simulink model "Plant"  (R2021b)
settings: Solver=VariableStepAuto  StartTime=0.0  StopTime=10.0  RelTol=1e-3
model workspace (MAT data in the model file):
  Ax = 0.000556
  Ay = 0.000556
  Az = 0.000635
  Ixx = 0.0075
  Iyy = 0.0075
  Izz = 0.013
  Jr = 6e-05
  b = 3.13e-05
  d = 7.5e-07
  g = 9.81
  l = 0.23
  m = 0.65
settings Model: Creator=aakas  LastModifiedBy=aakas

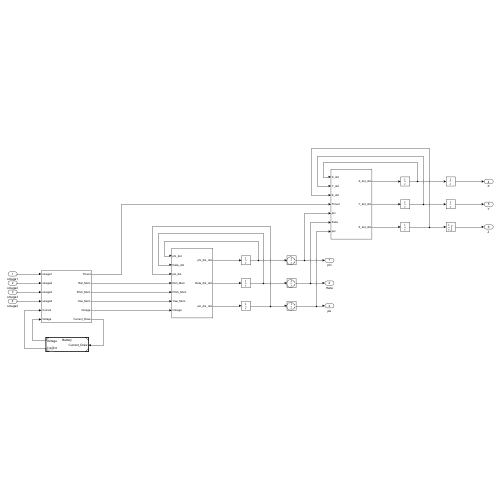
[thumbnail: Simulink's stored preview of the top-level diagram]
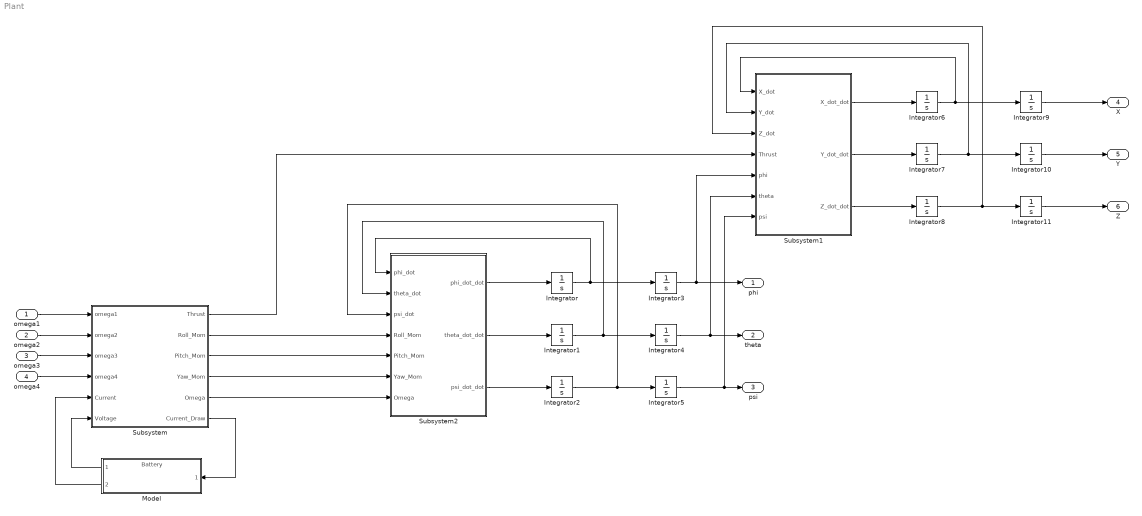
== system Plant ==
  omega1 : Inport
  omega2 : Inport  Port=2
  omega3 : Inport  Port=3
  omega4 : Inport  Port=4
  Integrator{,1..2,6..10} (8 alike) : Integrator
  Integrator11 : Integrator  LimitOutput=on  UpperSaturationLimit=0
  Integrator3 : Integrator  WrapState=on
  Integrator4 : Integrator  WrapState=on
  Integrator5 : Integrator  WrapState=on
  Model : ModelReference  ModelNameDialog=Battery.slx  SimulationMode=Normal  ModelReferenceVersion=1.8
  Subsystem : Subsystem
  Subsystem1 : Subsystem
  Subsystem2 : Subsystem
  phi : Outport
  theta : Outport  Port=2
  psi : Outport  Port=3
  X : Outport  Port=4
  Y : Outport  Port=5
  Z : Outport  Port=6
  wires:
  omega1/1 -> Subsystem/1(omega1)
  omega2/1 -> Subsystem/2(omega2)
  omega3/1 -> Subsystem/3(omega3)
  omega4/1 -> Subsystem/4(omega4)
  Integrator/1 -> Integrator3/1, Subsystem2/1(phi_dot)
  Integrator2/1 -> Subsystem2/3(psi_dot), Integrator5/1
  Integrator3/1 -> Subsystem1/5(phi), phi/1
  Integrator4/1 -> Subsystem1/6(theta), theta/1
  Integrator5/1 -> Subsystem1/7(psi), psi/1
  Integrator1/1 -> Subsystem2/2(theta_dot), Integrator4/1
  Subsystem/2(Roll_Mom) -> Subsystem2/4(Roll_Mom)
  Subsystem/3(Pitch_Mom) -> Subsystem2/5(Pitch_Mom)
  Subsystem/4(Yaw_Mom) -> Subsystem2/6(Yaw_Mom)
  Subsystem/5(Omega) -> Subsystem2/7(Omega)
  Subsystem2/1(phi_dot_dot) -> Integrator/1
  Subsystem2/2(theta_dot_dot) -> Integrator1/1
  Subsystem2/3(psi_dot_dot) -> Integrator2/1
  Integrator6/1 -> Integrator9/1, Subsystem1/1(X_dot)
  Integrator10/1 -> Y/1
  Integrator7/1 -> Subsystem1/2(Y_dot), Integrator10/1
  Integrator11/1 -> Z/1
  Subsystem1/2(Y_dot_dot) -> Integrator7/1
  Subsystem1/3(Z_dot_dot) -> Integrator8/1
  Subsystem1/1(X_dot_dot) -> Integrator6/1
  Integrator9/1 -> X/1
  Integrator8/1 -> Subsystem1/3(Z_dot), Integrator11/1
  Subsystem/1(Thrust) -> Subsystem1/4(Thrust)
  Subsystem/6(Current_Draw) -> Model/1
  Model/1 -> Subsystem/6(Voltage)
  Model/2 -> Subsystem/5(Current)

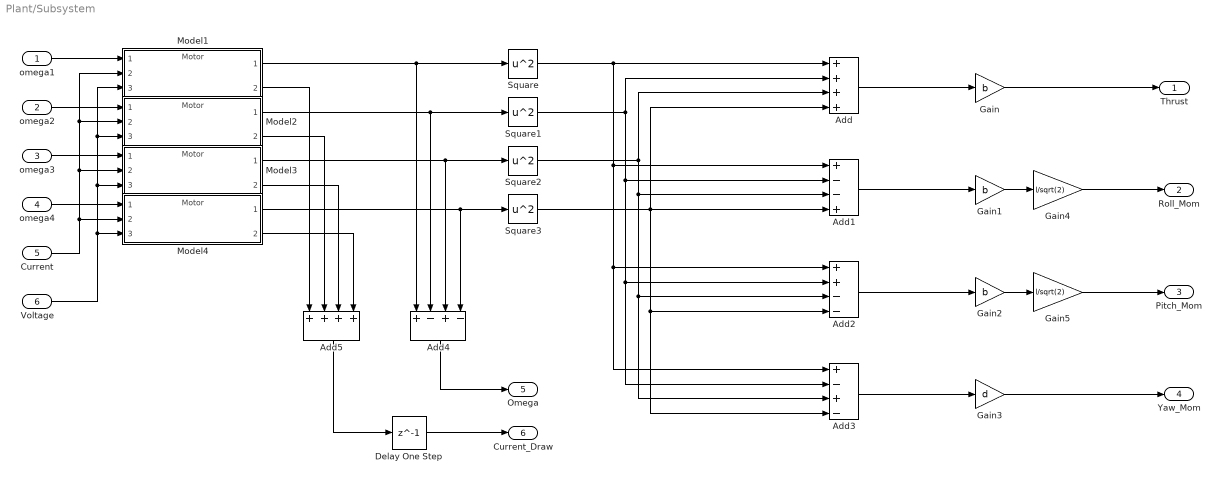
== system Plant/Subsystem ==
  omega1 : Inport
  omega2 : Inport  Port=2
  omega3 : Inport  Port=3
  omega4 : Inport  Port=4
  Current : Inport  Port=5
  Voltage : Inport  Port=6
  Add : Sum  Inputs=++++
  Add1 : Sum  Inputs=+--+
  Add2 : Sum  Inputs=++--
  Add3 : Sum  Inputs=+-+-
  Add4 : Sum  Inputs=+-+-
  Add5 : Sum  Inputs=++++
  Delay One Step : Delay  DelayLength=1
  Gain : Gain  Gain=b
  Gain1 : Gain  Gain=b
  Gain2 : Gain  Gain=b
  Gain3 : Gain  Gain=d
  Gain4 : Gain  Gain=l/sqrt(2)
  Gain5 : Gain  Gain=l/sqrt(2)
  Model{1..4} (4 alike) : ModelReference  ModelNameDialog=Motor.slx  SimulationMode=Normal  ModelReferenceVersion=1.6
  Square{,1..3} (4 alike) : Math  Operator=square  SaturateOnIntegerOverflow=on
  Thrust : Outport
  Roll_Mom : Outport  Port=2
  Pitch_Mom : Outport  Port=3
  Yaw_Mom : Outport  Port=4
  Omega : Outport  Port=5
  Current_Draw : Outport  Port=6
  wires:
  Add2/1 -> Gain2/1
  Model3/1 -> Add4/3, Square2/1
  Model4/1 -> Add4/4, Square3/1
  Add3/1 -> Gain3/1
  Gain2/1 -> Gain5/1
  Square2/1 -> Add3/3, Add2/3, Add1/3, Add/3
  Square3/1 -> Add3/4, Add2/4, Add1/4, Add/4
  Model2/1 -> Add4/2, Square1/1
  Add4/1 -> Omega/1
  Gain4/1 -> Roll_Mom/1
  Gain1/1 -> Gain4/1
  Model1/1 -> Add4/1, Square/1
  Square1/1 -> Add1/2, Add3/2, Add2/2, Add/2
  Gain3/1 -> Yaw_Mom/1
  Square/1 -> Add1/1, Add2/1, Add3/1, Add/1
  Add1/1 -> Gain1/1
  Add/1 -> Gain/1
  Gain/1 -> Thrust/1
  Gain5/1 -> Pitch_Mom/1
  omega1/1 -> Model1/1
  omega2/1 -> Model2/1
  omega3/1 -> Model3/1
  omega4/1 -> Model4/1
  Model1/2 -> Add5/1
  Model2/2 -> Add5/2
  Model4/2 -> Add5/4
  Model3/2 -> Add5/3
  Add5/1 -> Delay One Step/1
  Current/1 -> Model4/2, Model3/2, Model2/2, Model1/2
  Voltage/1 -> Model4/3, Model3/3, Model2/3, Model1/3
  Delay One Step/1 -> Current_Draw/1

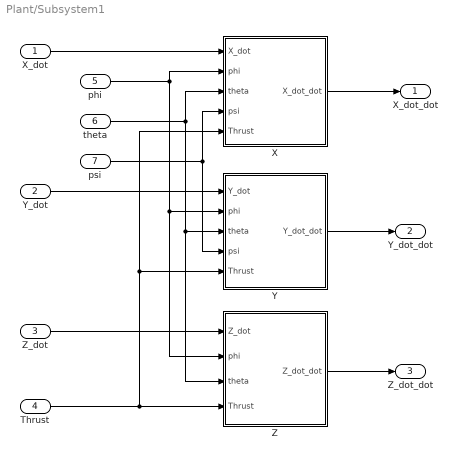
== system Plant/Subsystem1 ==
  X_dot : Inport
  Y_dot : Inport  Port=2
  Z_dot : Inport  Port=3
  Thrust : Inport  Port=4
  phi : Inport  Port=5
  theta : Inport  Port=6
  psi : Inport  Port=7
  X : Subsystem
  Y : Subsystem
  Z : Subsystem
  X_dot_dot : Outport
  Y_dot_dot : Outport  Port=2
  Z_dot_dot : Outport  Port=3
  wires:
  X/1(X_dot_dot) -> X_dot_dot/1
  Z/1(Z_dot_dot) -> Z_dot_dot/1
  Y/1(Y_dot_dot) -> Y_dot_dot/1
  X_dot/1 -> X/1(X_dot)
  Y_dot/1 -> Y/1(Y_dot)
  Z_dot/1 -> Z/1(Z_dot)
  phi/1 -> Z/2(phi), Y/2(phi), X/2(phi)
  theta/1 -> Z/3(theta), Y/3(theta), X/3(theta)
  psi/1 -> Y/4(psi), X/4(psi)
  Thrust/1 -> Z/4(Thrust), Y/5(Thrust), X/5(Thrust)

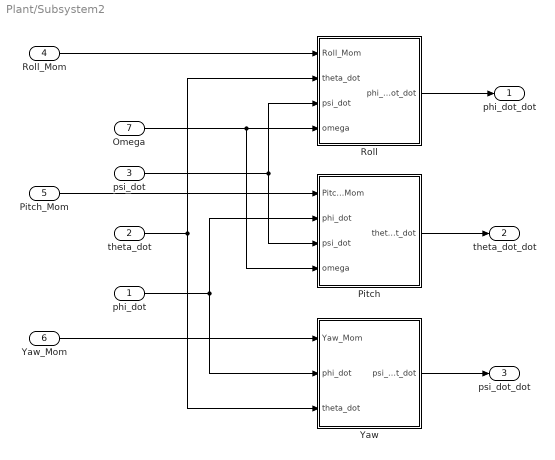
== system Plant/Subsystem2 ==
  phi_dot : Inport
  theta_dot : Inport  Port=2
  psi_dot : Inport  Port=3
  Roll_Mom : Inport  Port=4
  Pitch_Mom : Inport  Port=5
  Yaw_Mom : Inport  Port=6
  Omega : Inport  Port=7
  Pitch : Subsystem
  Roll : Subsystem
  Yaw : Subsystem
  phi_dot_dot : Outport
  theta_dot_dot : Outport  Port=2
  psi_dot_dot : Outport  Port=3
  wires:
  Roll/1(phi_dot_dot) -> phi_dot_dot/1
  Yaw/1(psi_dot_dot) -> psi_dot_dot/1
  Pitch/1(theta_dot_dot) -> theta_dot_dot/1
  Yaw_Mom/1 -> Yaw/1(Yaw_Mom)
  Roll_Mom/1 -> Roll/1(Roll_Mom)
  theta_dot/1 -> Yaw/3(theta_dot), Roll/2(theta_dot)
  Pitch_Mom/1 -> Pitch/1(Pitch_Mom)
  Omega/1 -> Pitch/4(omega), Roll/4(omega)
  psi_dot/1 -> Roll/3(psi_dot), Pitch/3(psi_dot)
  phi_dot/1 -> Yaw/2(phi_dot), Pitch/2(phi_dot)

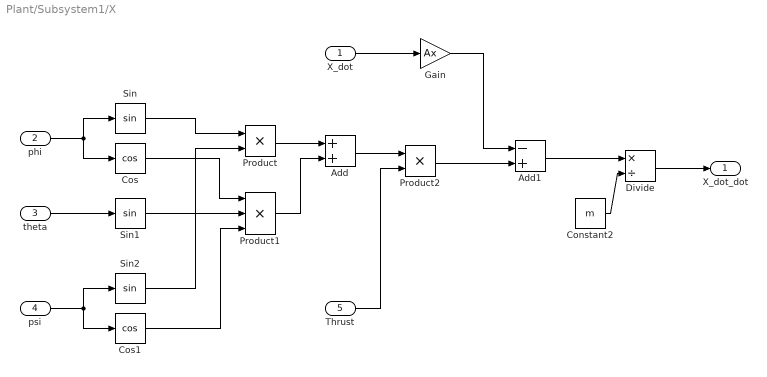
== system Plant/Subsystem1/X ==
  X_dot : Inport
  phi : Inport  Port=2
  theta : Inport  Port=3
  psi : Inport  Port=4
  Thrust : Inport  Port=5
  Add : Sum
  Add1 : Sum  Inputs=-+
  Constant2 : Constant  Value=m
  Cos : Trigonometry  Operator=cos
  Cos1 : Trigonometry  Operator=cos
  Divide : Product  Inputs=*/
  Gain : Gain  Gain=Ax
  Product : Product
  Product1 : Product  Inputs=3
  Product2 : Product
  Sin : Trigonometry
  Sin1 : Trigonometry
  Sin2 : Trigonometry
  X_dot_dot : Outport
  wires:
  Divide/1 -> X_dot_dot/1
  Constant2/1 -> Divide/2
  psi/1 -> Cos1/1, Sin2/1
  phi/1 -> Cos/1, Sin/1
  theta/1 -> Sin1/1
  Sin/1 -> Product/1
  Sin2/1 -> Product/2
  Cos/1 -> Product1/1
  Sin1/1 -> Product1/2
  Cos1/1 -> Product1/3
  Product/1 -> Add/1
  Product1/1 -> Add/2
  Add/1 -> Product2/1
  Thrust/1 -> Product2/2
  Product2/1 -> Add1/2
  Add1/1 -> Divide/1
  X_dot/1 -> Gain/1
  Gain/1 -> Add1/1

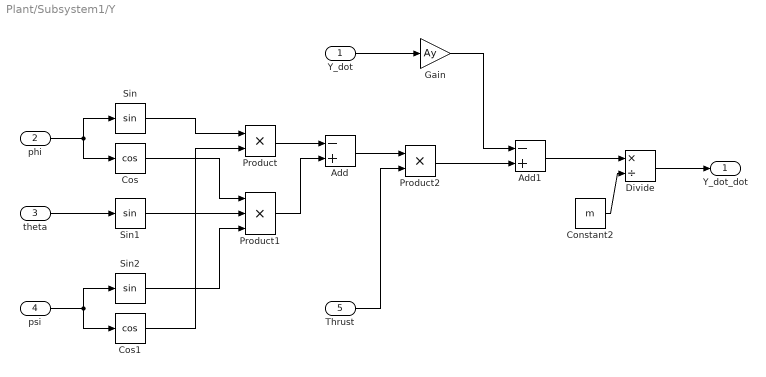
== system Plant/Subsystem1/Y ==
  Y_dot : Inport
  phi : Inport  Port=2
  theta : Inport  Port=3
  psi : Inport  Port=4
  Thrust : Inport  Port=5
  Add : Sum  Inputs=-+
  Add1 : Sum  Inputs=-+
  Constant2 : Constant  Value=m
  Cos : Trigonometry  Operator=cos
  Cos1 : Trigonometry  Operator=cos
  Divide : Product  Inputs=*/
  Gain : Gain  Gain=Ay
  Product : Product
  Product1 : Product  Inputs=3
  Product2 : Product
  Sin : Trigonometry
  Sin1 : Trigonometry
  Sin2 : Trigonometry
  Y_dot_dot : Outport
  wires:
  Add/1 -> Product2/1
  Cos/1 -> Product1/1
  theta/1 -> Sin1/1
  Sin2/1 -> Product1/3
  Cos1/1 -> Product/2
  Thrust/1 -> Product2/2
  Product1/1 -> Add/2
  Product/1 -> Add/1
  Product2/1 -> Add1/2
  Constant2/1 -> Divide/2
  Divide/1 -> Y_dot_dot/1
  phi/1 -> Cos/1, Sin/1
  Add1/1 -> Divide/1
  Gain/1 -> Add1/1
  Y_dot/1 -> Gain/1
  Sin/1 -> Product/1
  psi/1 -> Cos1/1, Sin2/1
  Sin1/1 -> Product1/2

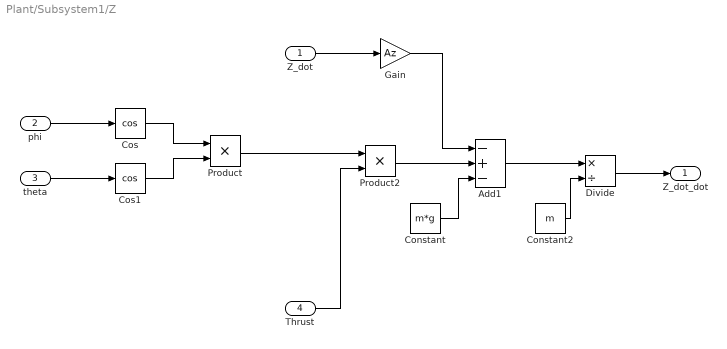
== system Plant/Subsystem1/Z ==
  Z_dot : Inport
  phi : Inport  Port=2
  theta : Inport  Port=3
  Thrust : Inport  Port=4
  Add1 : Sum  Inputs=-+-
  Constant : Constant  Value=m*g
  Constant2 : Constant  Value=m
  Cos : Trigonometry  Operator=cos
  Cos1 : Trigonometry  Operator=cos
  Divide : Product  Inputs=*/
  Gain : Gain  Gain=Az
  Product : Product
  Product2 : Product
  Z_dot_dot : Outport
  wires:
  Product/1 -> Product2/1
  Cos/1 -> Product/1
  theta/1 -> Cos1/1
  Thrust/1 -> Product2/2
  Product2/1 -> Add1/2
  Constant2/1 -> Divide/2
  Divide/1 -> Z_dot_dot/1
  phi/1 -> Cos/1
  Add1/1 -> Divide/1
  Gain/1 -> Add1/1
  Z_dot/1 -> Gain/1
  Cos1/1 -> Product/2
  Constant/1 -> Add1/3

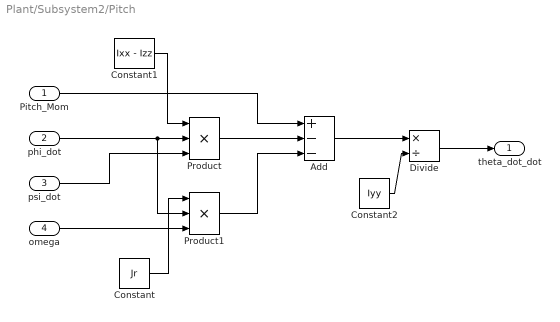
== system Plant/Subsystem2/Pitch ==
  Pitch_Mom : Inport
  phi_dot : Inport  Port=2
  psi_dot : Inport  Port=3
  omega : Inport  Port=4
  Add : Sum  Inputs=+--
  Constant : Constant  Value=Jr
  Constant1 : Constant  Value=Ixx - Izz
  Constant2 : Constant  Value=Iyy
  Divide : Product  Inputs=*/
  Product : Product  Inputs=3
  Product1 : Product  Inputs=3
  theta_dot_dot : Outport
  wires:
  Pitch_Mom/1 -> Add/1
  Constant1/1 -> Product/1
  Product/1 -> Add/2
  Constant/1 -> Product1/1
  Constant2/1 -> Divide/2
  Product1/1 -> Add/3
  psi_dot/1 -> Product/3
  Divide/1 -> theta_dot_dot/1
  Add/1 -> Divide/1
  phi_dot/1 -> Product/2, Product1/2
  omega/1 -> Product1/3

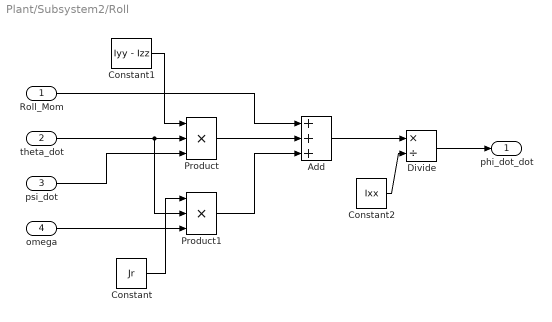
== system Plant/Subsystem2/Roll ==
  Roll_Mom : Inport
  theta_dot : Inport  Port=2
  psi_dot : Inport  Port=3
  omega : Inport  Port=4
  Add : Sum  Inputs=+++
  Constant : Constant  Value=Jr
  Constant1 : Constant  Value=Iyy - Izz
  Constant2 : Constant  Value=Ixx
  Divide : Product  Inputs=*/
  Product : Product  Inputs=3
  Product1 : Product  Inputs=3
  phi_dot_dot : Outport
  wires:
  Add/1 -> Divide/1
  Divide/1 -> phi_dot_dot/1
  omega/1 -> Product1/3
  theta_dot/1 -> Product/2, Product1/2
  Constant/1 -> Product1/1
  Constant1/1 -> Product/1
  psi_dot/1 -> Product/3
  Product/1 -> Add/2
  Product1/1 -> Add/3
  Roll_Mom/1 -> Add/1
  Constant2/1 -> Divide/2

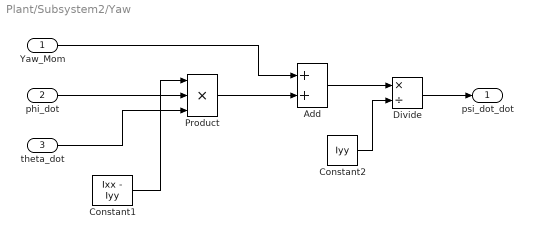
== system Plant/Subsystem2/Yaw ==
  Yaw_Mom : Inport
  phi_dot : Inport  Port=2
  theta_dot : Inport  Port=3
  Add : Sum
  Constant1 : Constant  Value=Ixx - Iyy
  Constant2 : Constant  Value=Iyy
  Divide : Product  Inputs=*/
  Product : Product  Inputs=3
  psi_dot_dot : Outport
  wires:
  phi_dot/1 -> Product/2
  Add/1 -> Divide/1
  Yaw_Mom/1 -> Add/1
  Product/1 -> Add/2
  Constant2/1 -> Divide/2
  Constant1/1 -> Product/1
  Divide/1 -> psi_dot_dot/1
  theta_dot/1 -> Product/3
